simulink model "ClutchControl_Overview"  (R2018a)
settings: Solver=VariableStepAuto  StartTime=0.0  StopTime=10.0  RelTol=1e-3
settings Model: Creator=rahul  LastModifiedBy=rahul

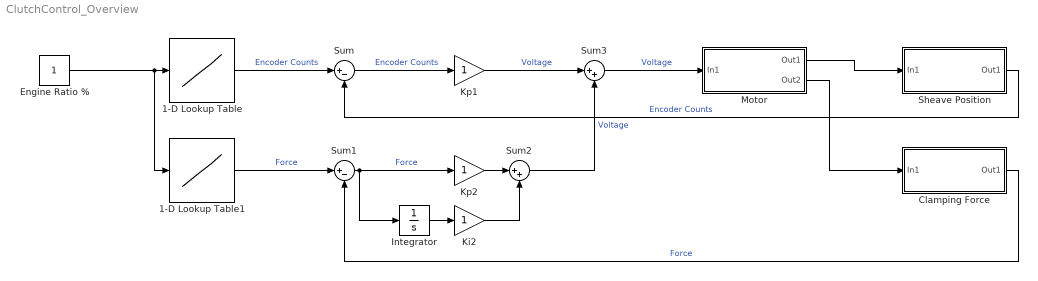
== system ClutchControl_Overview ==
  1-D Lookup Table : Lookup_n-D  NumberOfTableDimensions=1  BreakpointsForDimension1=[-5:5]  Table=tanh([-5:5])  InternalRulePriority=Speed  RndMeth=Simplest  InputSameDT=on
  1-D Lookup Table1 : Lookup_n-D  NumberOfTableDimensions=1  BreakpointsForDimension1=[-5:5]  Table=tanh([-5:5])  InternalRulePriority=Speed  RndMeth=Simplest  InputSameDT=on
  Clamping Force : Subsystem
  Engine Ratio % : Constant
  Integrator : Integrator
  Ki2 : Gain
  Kp1 : Gain
  Kp2 : Gain
  Motor : Subsystem
  Sheave Position : Subsystem
  Sum : Sum  Inputs=|+-
  Sum1 : Sum  Inputs=|+-
  Sum2 : Sum  Inputs=|++
  Sum3 : Sum  Inputs=|++
  wires:
  1-D Lookup Table/1 -> Sum/1  "Encoder Counts"
  1-D Lookup Table1/1 -> Sum1/1  "Force"
  Engine Ratio %/1 -> 1-D Lookup Table1/1, 1-D Lookup Table/1
  Motor/1(Out1) -> Sheave Position/1(In1)
  Sum/1 -> Kp1/1  "Encoder Counts"
  Integrator/1 -> Ki2/1
  Sum1/1 -> Integrator/1, Kp2/1  "Force"
  Kp2/1 -> Sum2/1
  Ki2/1 -> Sum2/2
  Sum2/1 -> Sum3/2  "Voltage"
  Kp1/1 -> Sum3/1  "Voltage"
  Sum3/1 -> Motor/1(In1)  "Voltage"
  Motor/2(Out2) -> Clamping Force/1(In1)
  Sheave Position/1(Out1) -> Sum/2  "Encoder Counts"
  Clamping Force/1(Out1) -> Sum1/2  "Force"

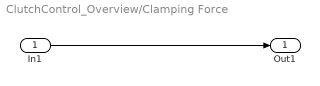
== system ClutchControl_Overview/Clamping Force ==
  In1 : Inport
  Out1 : Outport
  wires:
  In1/1 -> Out1/1

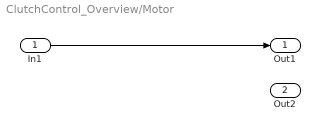
== system ClutchControl_Overview/Motor ==
  In1 : Inport
  Out1 : Outport
  Out2 : Outport  Port=2
  wires:
  In1/1 -> Out1/1

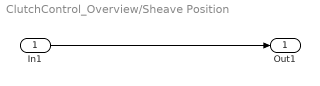
== system ClutchControl_Overview/Sheave Position ==
  In1 : Inport
  Out1 : Outport
  wires:
  In1/1 -> Out1/1
